simulink model "smith_praediktor"  (R2023a)
settings: Solver=VariableStepAuto  StartTime=0.0  StopTime=10.0  RelTol=1e-3
undefined symbols (not defined in the file or in its folder): vq_P1D
libraries: cstblocks x2, slident x1
settings Model: Creator=proto  LastModifiedBy=proto

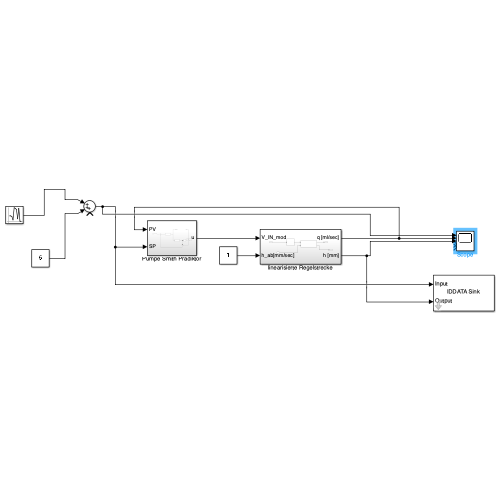
[thumbnail: Simulink's stored preview of the top-level diagram]
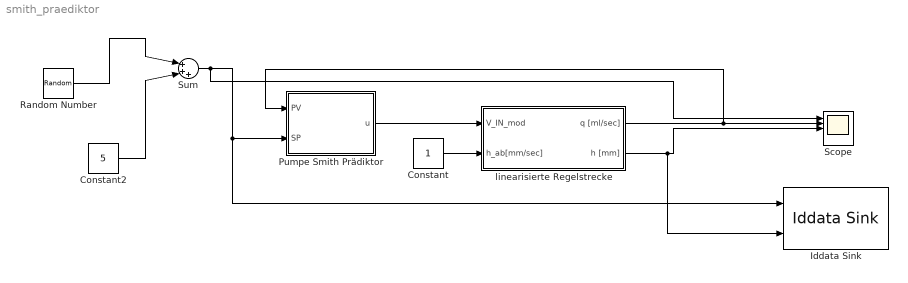
== system smith_praediktor ==
  Constant : Constant
  Constant2 : Constant  Value=5
  Iddata Sink : slident/Iddata Sink  datasetname=smith_data  Ts=0.1  isu=on  isy=on
  Pumpe Smith Prädiktor : Subsystem
  Random Number : RandomNumber  Mean=5  Variance=5  SampleTime=0.1
  Scope : Scope  NumInputPorts=5
  Sum : Sum  Inputs=|+++
  linearisierte Regelstrecke : Subsystem
  wires:
  linearisierte Regelstrecke/1(q [ml/sec]) -> Pumpe Smith Prädiktor/1(PV), Scope/2
  linearisierte Regelstrecke/2(h [mm]) -> Iddata Sink/2, Scope/3
  Sum/1 -> Scope/1, Iddata Sink/1, Pumpe Smith Prädiktor/2(SP)
  Pumpe Smith Prädiktor/1(u) -> linearisierte Regelstrecke/1(V_IN_mod)
  Constant/1 -> linearisierte Regelstrecke/2(h_ab[mm/sec])
  Constant2/1 -> Sum/2
  Random Number/1 -> Sum/1

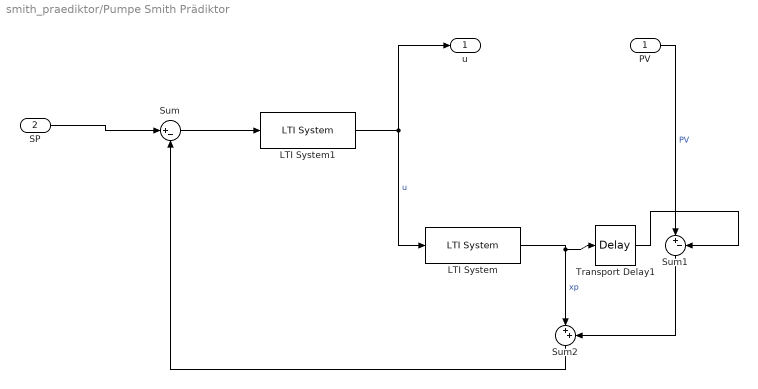
== system smith_praediktor/Pumpe Smith Prädiktor ==
  PV : Inport
  SP : Inport  Port=2
  LTI System : cstblocks/LTI System  sys=delay_free  IC=[]
  LTI System1 : cstblocks/LTI System  sys=delay_free_C  IC=[]
  Sum : Sum  Inputs=|+-
  Sum1 : Sum  Inputs=|+-
  Sum2 : Sum  Inputs=|++
  Transport Delay1 : TransportDelay  DelayTime=vq_P1D.Td
  u : Outport
  wires:
  PV/1 -> Sum1/1  "PV"
  SP/1 -> Sum/1
  Sum2/1 -> Sum/2
  Sum1/1 -> Sum2/2
  LTI System1/1 -> u/1, LTI System/1  "u"
  LTI System/1 -> Transport Delay1/1, Sum2/1  "xp"
  Transport Delay1/1 -> Sum1/2
  Sum/1 -> LTI System1/1

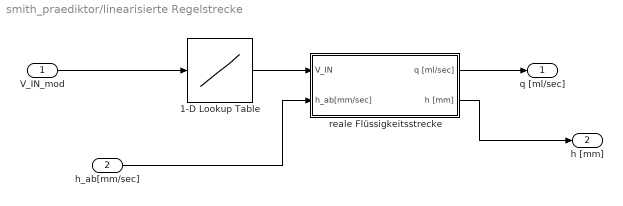
== system smith_praediktor/linearisierte Regelstrecke ==
  V_IN_mod : Inport
  h_ab[mm/sec] : Inport  Port=2
  1-D Lookup Table : Lookup_n-D  NumberOfTableDimensions=1  BreakpointsForDimension1=[-11.6,-10.1,-9.0,-7.65,-6.15,-4.4,-2.65,-0.01,0.01,2.65,4.4,6.15,7.65,9.0,10.1,11.6]  Table=[-10,-9,-8,-7,-6,-5,-4,-3,3,4,5,6,7,8,9,10]  InternalRulePriority=Speed  RndMeth=Simplest
  reale Flüssigkeitsstrecke : Subsystem
  q [ml/sec] : Outport
  h [mm] : Outport  Port=2
  wires:
  reale Flüssigkeitsstrecke/2(h [mm]) -> h [mm]/1
  V_IN_mod/1 -> 1-D Lookup Table/1
  reale Flüssigkeitsstrecke/1(q [ml/sec]) -> q [ml/sec]/1
  h_ab[mm/sec]/1 -> reale Flüssigkeitsstrecke/2(h_ab[mm/sec])
  1-D Lookup Table/1 -> reale Flüssigkeitsstrecke/1(V_IN)

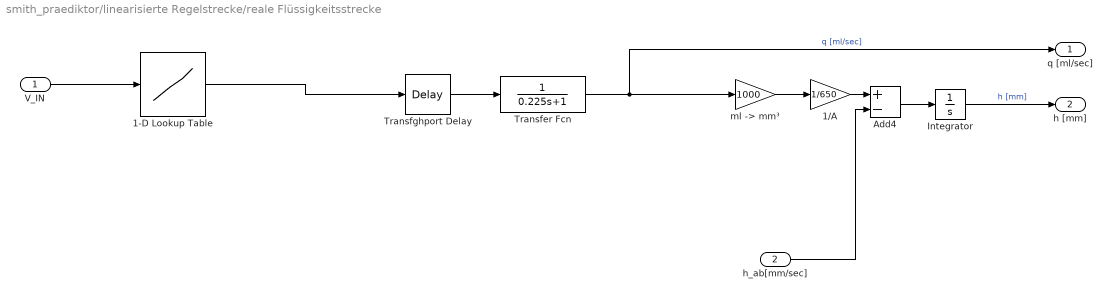
== system smith_praediktor/linearisierte Regelstrecke/reale Flüssigkeitsstrecke ==
  V_IN : Inport
  h_ab[mm/sec] : Inport  Port=2
  1-D Lookup Table : Lookup_n-D  NumberOfTableDimensions=1  BreakpointsForDimension1=[-10,-9,-8,-7,-6,-5,-4,-3,3,4,5,6,7,8,9,10]  Table=[-11.6,-10.1,-9.0,-7.65,-6.15,-4.4,-2.65,0,0,2.65,4.4,6.15,7.65,9.0,10.1,11.6]  InternalRulePriority=Speed  RndMeth=Simplest
  1/A : Gain  Gain=1/650
  Add4 : Sum  Inputs=+-
  Integrator : Integrator  InitialCondition=70  LimitOutput=on  UpperSaturationLimit=153  LowerSaturationLimit=0
  Transfer Fcn : TransferFcn  Denominator=[0.225 1]
  Transfghport Delay : TransportDelay  DelayTime=0.25
  "ml -> mm³" : Gain  Gain=1000
  q [ml/sec] : Outport
  h [mm] : Outport  Port=2
  wires:
  h_ab[mm/sec]/1 -> Add4/2
  V_IN/1 -> 1-D Lookup Table/1
  Integrator/1 -> h [mm]/1  "h [mm]"
  "ml -> mm³"/1 -> 1/A/1
  1-D Lookup Table/1 -> Transfghport Delay/1
  Transfghport Delay/1 -> Transfer Fcn/1
  1/A/1 -> Add4/1
  Transfer Fcn/1 -> q [ml/sec]/1, "ml -> mm³"/1  "q [ml/sec]"
  Add4/1 -> Integrator/1
